simulink model "cyo"  (R2025a)
settings: Solver=VariableStepAuto  StartTime=0.0  StopTime=10.0  RelTol=1e-3
undefined symbols (not defined in the file or in its folder): x_e

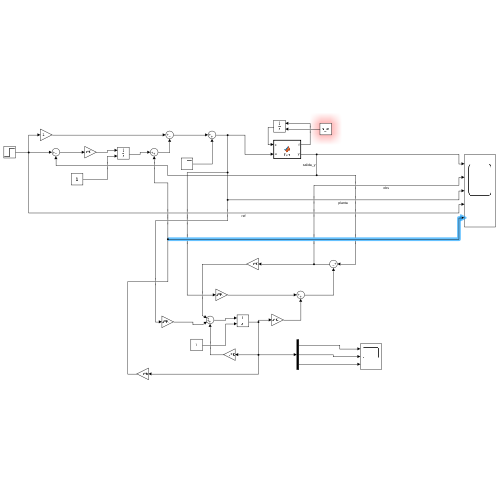
[thumbnail: Simulink's stored preview of the top-level diagram]
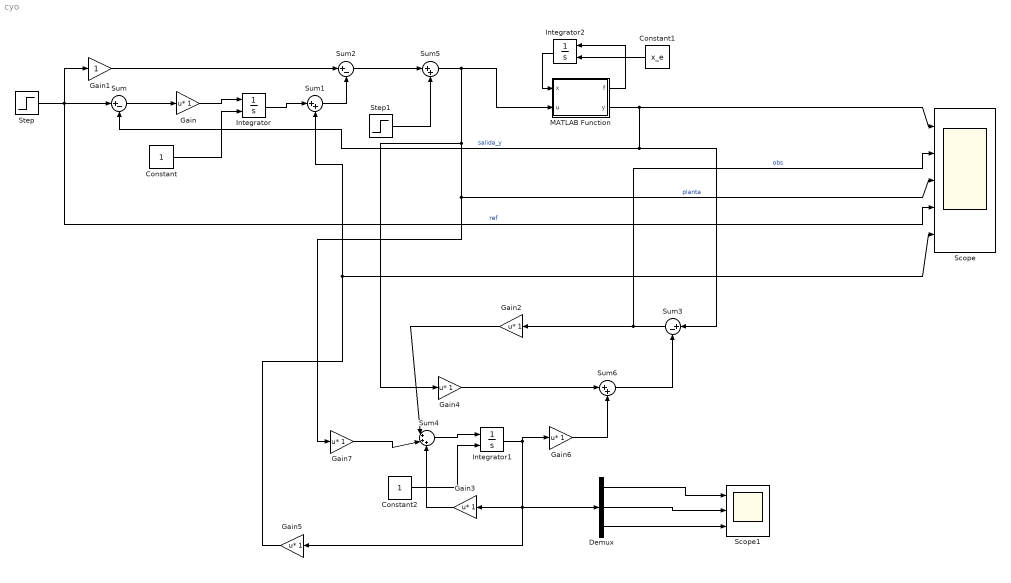
== system cyo ==
  Constant : Constant
  Constant1 : Constant  Value=x_e  VectorParams1D=off
  Constant2 : Constant
  Demux : Demux  Outputs=3
  Gain{,2..7} (7 alike) : Gain  Multiplication=Matrix(u*K)
  Gain1 : Gain
  Integrator : Integrator  InitialConditionSource=external
  Integrator1 : Integrator  InitialConditionSource=external
  Integrator2 : Integrator  InitialConditionSource=external
  MATLAB Function : MATLAB Function  TreatAsAtomicUnit=on
  Scope : Scope  NumInputPorts=5
  Scope1 : Scope  NumInputPorts=3
  Step : Step  SampleTime=0
  Step1 : Step  SampleTime=0
  Sum : Sum  Inputs=|+-
  Sum1 : Sum  Inputs=|++
  Sum2 : Sum  Inputs=|+-
  Sum3 : Sum  Inputs=|+-
  Sum4 : Sum  Inputs=|+++
  Sum5 : Sum  Inputs=|++
  Sum6 : Sum  Inputs=|++
  wires:
  Sum/1 -> Gain/1
  Integrator/1 -> Sum1/1
  Gain/1 -> Integrator/1
  Gain1/1 -> Sum2/1
  Sum1/1 -> Sum2/2
  Sum2/1 -> Sum5/1
  Step1/1 -> Sum5/2
  Integrator1/1 -> Gain6/1, Demux/1, Gain5/1, Gain3/1
  Gain6/1 -> Sum6/2
  Gain4/1 -> Sum6/1
  Sum6/1 -> Sum3/2
  Sum4/1 -> Integrator1/1
  Gain2/1 -> Sum4/1
  Gain3/1 -> Sum4/3
  Gain7/1 -> Sum4/2
  Demux/1 -> Scope1/1
  Demux/2 -> Scope1/2
  Demux/3 -> Scope1/3
  MATLAB Function/2(y) -> Sum/2, Sum3/1, Scope/1  "salida_y"
  Integrator2/1 -> MATLAB Function/1(x)
  Constant1/1 -> Integrator2/2
  Constant/1 -> Integrator/2
  MATLAB Function/1(f) -> Integrator2/1
  Constant2/1 -> Integrator1/2
  Gain5/1 -> Sum1/2, Scope/5
  Sum3/1 -> Gain2/1, Scope/2  "obs"
  Step/1 -> Gain1/1, Scope/4, Sum/1  "ref"
  Sum5/1 -> Scope/3, Gain7/1, Gain4/1, MATLAB Function/2(u)  "planta"

== matlab function cyo/MATLAB Function ==
  data: f output; x input; u input; y output
function [f,y] = fcn(x,u)
x=[x1;x2;x3]

g=10;
m=0.1;
L=1e-2;
R=4;

f1 = x(2);
f2 = g-x(3)*/(m*x(1));
f3 = u/L-x(3)*R/L;

f=[f1;f2;f3];

y = x(1);
